simulink model "FIR_filterTestManual"  (R2019a)
settings: Solver=VariableStepAuto  StartTime=0.0  StopTime=10.0  RelTol=1e-3
values from neighbouring files (symbols this model uses):
  Ts = 1/Fs    (= 2.08333333333e-05)    [FIR_filterTestm.m]    (also in JMAP_INIT.m; blockVerification.m; block_verScript.m; ksi_verScript.m)
libraries: simulink x2, hdlsllib x2, dsphdlfiltering x2
settings Model: Creator=Showi  LastModifiedBy=Showi

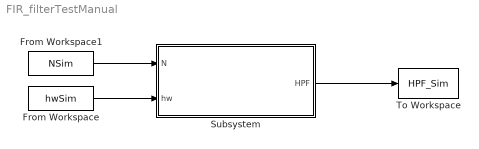
== system FIR_filterTestManual ==
  From Workspace : FromWorkspace  VariableName=hwSim  SampleTime=Ts
  From Workspace1 : FromWorkspace  VariableName=NSim  SampleTime=Ts
  Subsystem : Subsystem
  To Workspace : ToWorkspace  VariableName=HPF_Sim  SaveFormat=Structure With Time  SampleTime=-1
  wires:
  Subsystem/1(HPF) -> To Workspace/1
  From Workspace/1 -> Subsystem/2(hw)
  From Workspace1/1 -> Subsystem/1(N)

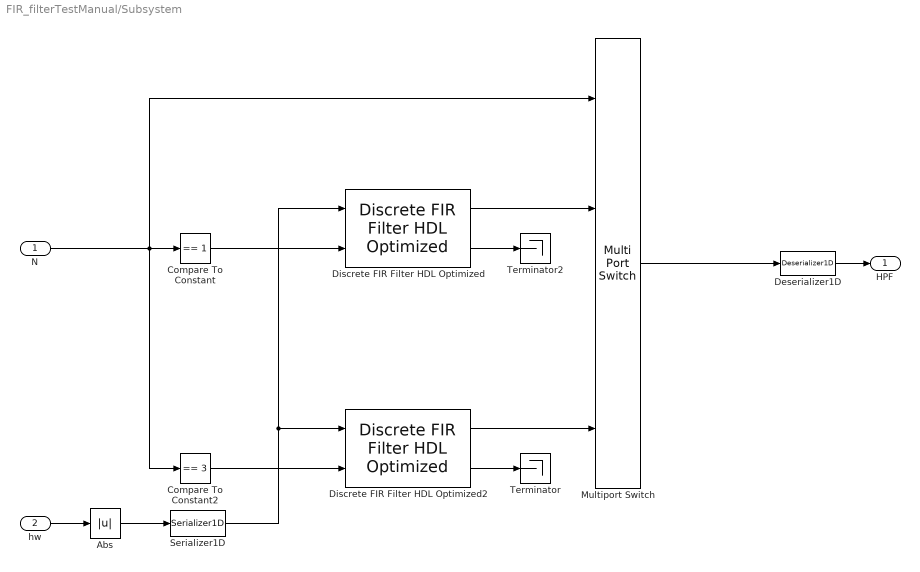
== system FIR_filterTestManual/Subsystem ==
  N : Inport
  hw : Inport  Port=2
  Abs : Abs
  Compare To Constant : simulink/Logic and Bit Operations/Compare To Constant  relop===  const=1  OutDataTypeStr=boolean
  Compare To Constant2 : simulink/Logic and Bit Operations/Compare To Constant  relop===  const=3  OutDataTypeStr=boolean
  Deserializer1D : hdlsllib/HDL Operations/Deserializer1D  Ratio=FFT_size  IdleCycles=0  InitialCondition=0  startIn=off  validIn=off  validOut=off  inputDataDimensions=-1  inputSampleTime=-1  inputSignalType=auto
      settings: SourceProductName=Simulink  SourceProductBaseCode=SL
  Discrete FIR Filter HDL Optimized : dsphdlfiltering/Discrete FIR Filter HDL Optimized  NumeratorSource=Property  Numerator=[1, 0, 0]  NumeratorPrototype=[1, 0, 0]  FilterStructure=Direct form systolic  SerializationOption=Minimum number of cycles between valid input samples  NumberOfCycles=2  NumberOfMultipliers=2  SimulateUsing=Code generation  roundingMode=Floor  overflowMode=off  CoefficientsDataTypeStr=Inherit: Same word length as input  CoefficientsMin=[]  CoefficientsMax=[]  OutputMin=[]  OutputMax=[]  ResetInputPort=off  HDLGlobalReset=off
      settings: SourceProductName=DSP System Toolbox  SourceProductBaseCode=DS
  Discrete FIR Filter HDL Optimized2 : dsphdlfiltering/Discrete FIR Filter HDL Optimized  NumeratorSource=Property  Numerator=[1/3, 1/3, 1/3]  NumeratorPrototype=[ 0.5, 0.5 ]  FilterStructure=Direct form systolic  SerializationOption=Minimum number of cycles between valid input samples  NumberOfCycles=2  NumberOfMultipliers=2  SimulateUsing=Code generation  roundingMode=Floor  overflowMode=off  CoefficientsDataTypeStr=Inherit: Same word length as input  CoefficientsMin=[]  CoefficientsMax=[]  OutputMin=[]  OutputMax=[]  ResetInputPort=off  HDLGlobalReset=off
      settings: SourceProductName=DSP System Toolbox  SourceProductBaseCode=DS
  Multiport Switch : MultiPortSwitch
  Serializer1D : hdlsllib/HDL Operations/Serializer1D  Ratio=FFT_size  IdleCycles=0  validIn=off  startOut=off  validOut=off  inputDataDimensions=-1  inputSampleTime=-1  inputSignalType=auto
      settings: SourceProductName=Simulink  SourceProductBaseCode=SL
  Terminator : Terminator
  Terminator2 : Terminator
  HPF : Outport
  wires:
  N/1 -> Multiport Switch/1, Compare To Constant2/1, Compare To Constant/1
  hw/1 -> Abs/1
  Compare To Constant/1 -> Discrete FIR Filter HDL Optimized/2
  Compare To Constant2/1 -> Discrete FIR Filter HDL Optimized2/2
  Discrete FIR Filter HDL Optimized2/2 -> Terminator/1
  Discrete FIR Filter HDL Optimized/2 -> Terminator2/1
  Abs/1 -> Serializer1D/1
  Multiport Switch/1 -> Deserializer1D/1
  Serializer1D/1 -> Discrete FIR Filter HDL Optimized/1, Discrete FIR Filter HDL Optimized2/1
  Discrete FIR Filter HDL Optimized2/1 -> Multiport Switch/4
  Discrete FIR Filter HDL Optimized/1 -> Multiport Switch/2
  Deserializer1D/1 -> HPF/1
